simulink model "project"  (R2016a)
settings: Solver=VariableStepAuto  SolverMode=SingleTasking  StartTime=0.0  StopTime=10.0  RelTol=1e-3
libraries: fuzblock x1
settings Model: Creator=MATREX  LastModifiedBy=MATREX
settings DataIOCC: LimitDataPoints=on  SaveOutput=off  SaveTime=off
settings OptimizationCC: BlockReduction=off  BooleanDataType=off
settings DebuggingCC: SaveWithParameterizedLinksMsg=none  UnderspecifiedInitializationDetection=Classic  MergeDetectMultiDrivingBlocksExec=none  SignalResolutionControl=TryResolveAllWithWarning  AllowSymbolicDim=off
settings HardwareCC: TargetUnknown=on

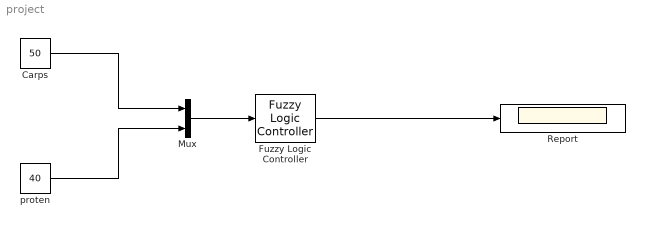
== system project ==
  Carps : Constant  Value=50
  Fuzzy Logic Controller : fuzblock/Fuzzy Logic  Controller  fis=['project.fis']
  Mux : Mux  Inputs=2
  Report : Scope
  proten : Constant  Value=40
  wires:
  Fuzzy Logic Controller/1 -> Report/1
  Mux/1 -> Fuzzy Logic Controller/1
  Carps/1 -> Mux/1
  proten/1 -> Mux/2
